simulink model "task_9_model"  (R2020a)
settings: Solver=VariableStepAuto  StartTime=0.0  StopTime=10  RelTol=1e-3
values from neighbouring files (symbols this model uses):
  h = 1    [task_6.m]    (also in task_8.m; task_9.m)
  K_Psi = K    [task_9.m]
  K_w = K    [task_9.m]
  L = 1    [task_6.m]    (also in task_8.m; task_9.m)
  R = 1    [task_6.m]    (also in task_8.m; task_9.m)
  theta_ref = pi/4    (= 0.785398163397)    [task_6.m]    (also in task_9.m)
  x_ref = 1    [task_9.m]
  y_ref = 1    [task_9.m]
settings Model: Creator=jryl9  LastModifiedBy=jryl9

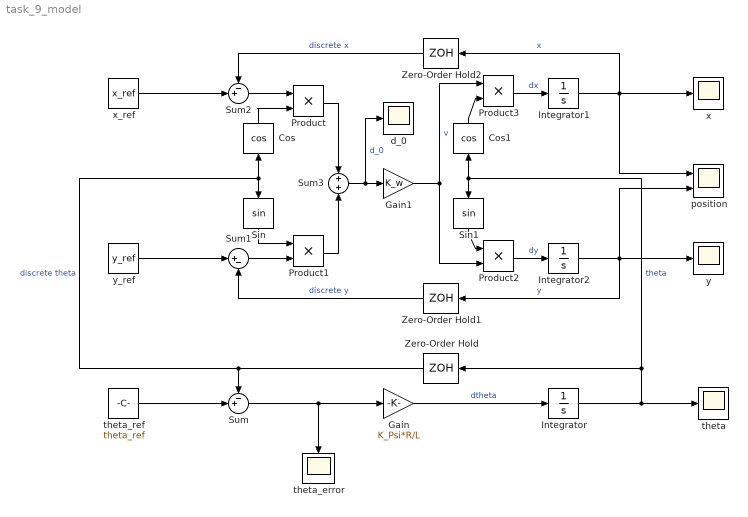
== system task_9_model ==
  Cos : Trigonometry  Operator=cos
  Cos1 : Trigonometry  Operator=cos
  Gain : Gain  Gain=K_Psi*R/L
  Gain1 : Gain  Gain=K_w
  Integrator : Integrator
  Integrator1 : Integrator
  Integrator2 : Integrator
  Product{,1..3} (4 alike) : Product
  Sin : Trigonometry
  Sin1 : Trigonometry
  Sum : Sum  Inputs=-+|
  Sum1 : Sum  Inputs=|+-
  Sum2 : Sum  Inputs=-+|
  Sum3 : Sum  Inputs=+|+
  Zero-Order Hold : ZeroOrderHold  SampleTime=h
  Zero-Order Hold1 : ZeroOrderHold  SampleTime=h
  Zero-Order Hold2 : ZeroOrderHold  SampleTime=h
  d_0 : Scope
  position : Scope  NumInputPorts=2
  theta : Scope
  theta_error : Scope
  theta_ref : Constant  Value=theta_ref
  x : Scope
  x_ref : Constant  Value=x_ref
  y : Scope
  y_ref : Constant  Value=y_ref
  wires:
  Sum/1 -> theta_error/1, Gain/1
  Gain/1 -> Integrator/1  "dtheta"
  Integrator/1 -> theta/1, Sin1/1, Cos1/1, Zero-Order Hold/1  "theta"
  theta_ref/1 -> Sum/2
  Sum3/1 -> d_0/1, Gain1/1  "d_0"
  Sum2/1 -> Product/1
  Sum1/1 -> Product1/2
  Gain1/1 -> Product3/1, Product2/2  "v"
  y_ref/1 -> Sum1/1
  Product1/1 -> Sum3/2
  Product/1 -> Sum3/1
  Integrator2/1 -> y/1, position/2, Zero-Order Hold1/1  "y"
  Integrator1/1 -> x/1, position/1, Zero-Order Hold2/1  "x"
  Zero-Order Hold/1 -> Sum/1, Sin/1, Cos/1  "discrete theta"
  x_ref/1 -> Sum2/2
  Zero-Order Hold1/1 -> Sum1/2  "discrete y"
  Zero-Order Hold2/1 -> Sum2/1  "discrete x"
  Cos/1 -> Product/2
  Sin/1 -> Product1/1
  Product2/1 -> Integrator2/1  "dy"
  Product3/1 -> Integrator1/1  "dx"
  Cos1/1 -> Product3/2
  Sin1/1 -> Product2/1
